simulink model "qft_sim"  (Simulink 5.0)
settings: Solver=ode45  StartTime=0.0  StopTime=0.20  RelTol=1e-3
values from neighbouring files (symbols this model uses):
  denF = df0    [qftex2_app.m]
  numF = nf0    (= 150)    [qftex2_app.m]
undefined symbols (not defined in the file or in its folder): denG, numG
libraries: simulink x1
settings Model: LastModifiedBy=Administrator  ExtModeTrigMode=oneshot  ExtModeArmWhenConnect=off  LimitDataPoints=off  BooleanDataType=off

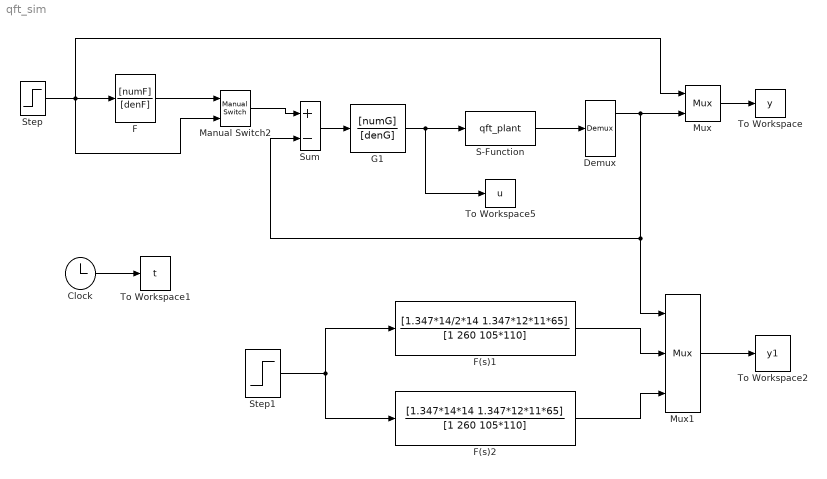
== system qft_sim ==
  Clock : Clock
      settings: Decimation=10
  Demux : Demux  Outputs=2
  F : TransferFcn  Numerator=[numF]  Denominator=[denF]
  F(s)1 : TransferFcn  Numerator=[1.347*14/2*14 1.347*12*11*65]  Denominator=[1 260 105*110]
  F(s)2 : TransferFcn  Numerator=[1.347*14*14 1.347*12*11*65]  Denominator=[1 260 105*110]
  G1 : TransferFcn  Numerator=[numG]  Denominator=[denG]
  Manual Switch2 : simulink/Signal Routing/Manual Switch  sw=0  action=0
  Mux : Mux  Inputs=2
  Mux1 : Mux  Inputs=3
  S-Function : S-Function  FunctionName=qft_plant
  Step : Step  Time=0  SampleTime=0
  Step1 : Step  Time=0  SampleTime=0
  Sum : Sum  Inputs=+-  SaturateOnIntegerOverflow=on  InputSameDT=on
  To Workspace : ToWorkspace  VariableName=y  SampleTime=-1  SaveFormat=Array
  To Workspace1 : ToWorkspace  VariableName=t  SampleTime=-1  SaveFormat=Array
  To Workspace2 : ToWorkspace  VariableName=y1  SampleTime=-1  SaveFormat=Array
  To Workspace5 : ToWorkspace  VariableName=u  SampleTime=-1  SaveFormat=Array
  wires:
  S-Function/1 -> Demux/1
  Clock/1 -> To Workspace1/1
  Step/1 -> Mux/1, F/1, Manual Switch2/2
  Manual Switch2/1 -> Sum/1
  Sum/1 -> G1/1
  F/1 -> Manual Switch2/1
  Demux/1 -> Mux/2, Sum/2, Mux1/1
  Mux/1 -> To Workspace/1
  Step1/1 -> F(s)1/1, F(s)2/1
  Mux1/1 -> To Workspace2/1
  F(s)1/1 -> Mux1/2
  F(s)2/1 -> Mux1/3
  G1/1 -> S-Function/1, To Workspace5/1
